simulink model "Adder"  (R2023b)
settings: Solver=VariableStepAuto  StartTime=0.0  StopTime=10.0  RelTol=1e-3
model workspace (MAT data in the model file):
  A = 2
  B = 1
settings Model: Creator=kapis  LastModifiedBy=kapis

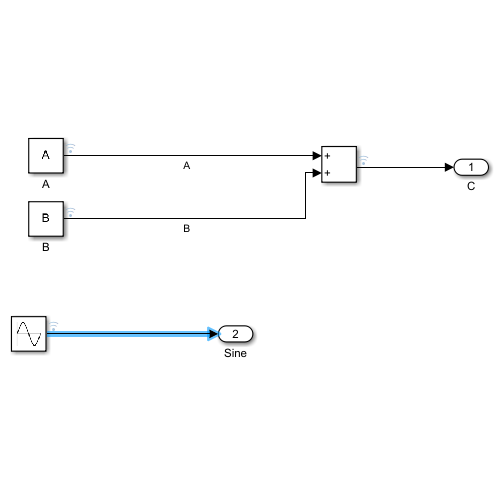
[thumbnail: Simulink's stored preview of the top-level diagram]
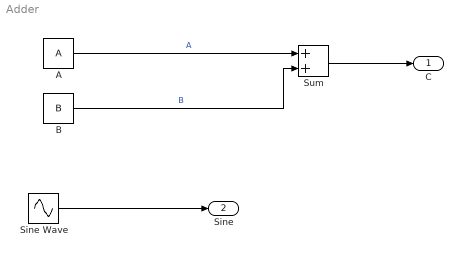
== system Adder ==
  A : Constant  Value=A
  B : Constant  Value=B
  Sine Wave : Sin  SampleTime=0
  Sum : Sum
  C : Outport
  Sine : Outport  Port=2
  wires:
  Sum/1 -> C/1
  A/1 -> Sum/1  "A"
  B/1 -> Sum/2  "B"
  Sine Wave/1 -> Sine/1
